simulink model "Incrementor_4BIT"  (R2018a)
settings: Solver=VariableStepAuto  StartTime=0.0  StopTime=10.0  RelTol=1e-3
settings Model: Creator=midog  LastModifiedBy=midog

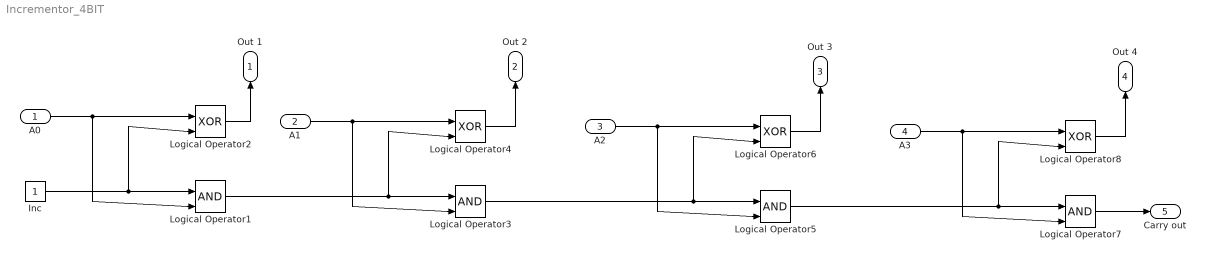
== system Incrementor_4BIT ==
  A0 : Inport  OutDataTypeStr=boolean
  A1 : Inport  Port=2
  A2 : Inport  Port=3
  A3 : Inport  Port=4
  Inc : Constant  OutDataTypeStr=boolean
  Logical Operator{1,3,5,7} (4 alike) : Logic  IconShape=distinctive  AllPortsSameDT=off  OutDataTypeStr=boolean
  Logical Operator{2,4,6,8} (4 alike) : Logic  Operator=XOR  IconShape=distinctive  AllPortsSameDT=off  OutDataTypeStr=boolean
  Out 1 : Outport
  Out 2 : Outport  Port=2
  Out 3 : Outport  Port=3
  Out 4 : Outport  Port=4
  Carry out : Outport  Port=5
  wires:
  Logical Operator2/1 -> Out 1/1
  Inc/1 -> Logical Operator2/2, Logical Operator1/1
  A0/1 -> Logical Operator1/2, Logical Operator2/1
  Logical Operator4/1 -> Out 2/1
  Logical Operator1/1 -> Logical Operator4/2, Logical Operator3/1
  A1/1 -> Logical Operator3/2, Logical Operator4/1
  A2/1 -> Logical Operator5/2, Logical Operator6/1
  Logical Operator3/1 -> Logical Operator6/2, Logical Operator5/1
  Logical Operator6/1 -> Out 3/1
  A3/1 -> Logical Operator7/2, Logical Operator8/1
  Logical Operator7/1 -> Carry out/1
  Logical Operator5/1 -> Logical Operator8/2, Logical Operator7/1
  Logical Operator8/1 -> Out 4/1
